simulink model "SingleEcho"  (R2020a)
settings: Solver=VariableStepAuto  StartTime=0.0  StopTime=1000000  RelTol=1e-3
libraries: audiosources x1, dspsnks4 x1
settings Model: Creator=ace  LastModifiedBy=ace

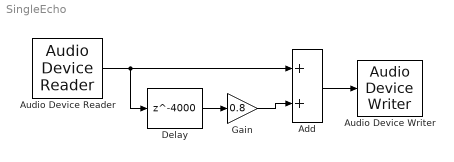
== system SingleEcho ==
  Add : Sum
  Audio Device Reader : audiosources/Audio Device Reader  Driver=CoreAudio  Device=Default  SampleRate=8000  NumChannels=1  SamplesPerFrame=64  BitDepth=16-bit integer  NumBuffers=10  DefaultInputChannelMapping=on  InputChannelMapping=1:2  OutputNumOverrunSamples=off  OutputDataType=double  DriverIdx=5  DeviceWarnFlag=''
      settings: SourceProductBaseCode=AU
  Audio Device Writer : dspsnks4/Audio Device Writer  Driver=CoreAudio  Device=Default  InheritSampleRate=on  SampleRate=44100  BitDepth=16-bit integer  BufferSize=4096  NumBuffers=10  DefaultOutputChannelMapping=on  OutputChannelMapping=1:2  OutputNumUnderrunSamples=off  DriverIdx=5  DeviceWarnFlag=''
  Delay : Delay  DelayLength=4000  InputProcessing=Columns as channels (frame based)
  Gain : Gain  Gain=0.8
  wires:
  Delay/1 -> Gain/1
  Gain/1 -> Add/2
  Audio Device Reader/1 -> Delay/1, Add/1
  Add/1 -> Audio Device Writer/1
